simulink model "rcos_1"  (R2019b)
settings: Solver=VariableStepAuto  StartTime=0.0  StopTime=5e-3  RelTol=1e-3
values from neighbouring files (symbols this model uses):
  filter = rcosdesign(alpha,symNum,sym,'sqrt')    [loopFil.m]
libraries: dspsrcs4 x1
settings Model: Creator=Administrator  LastModifiedBy=Administrator

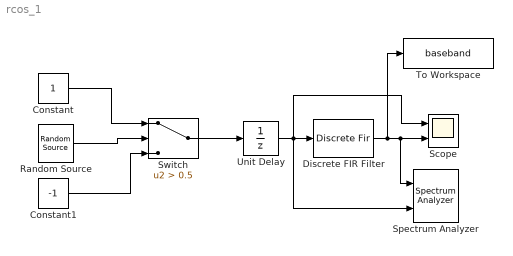
== system rcos_1 ==
  Constant : Constant  SampleTime=1/(6*19.2e3)
  Constant1 : Constant  Value=-1  SampleTime=1/(6*19.2e3)
  Discrete FIR Filter : DiscreteFir  Coefficients=filter(2,:)
  Random Source : dspsrcs4/Random Source  SrcType=Uniform  NormMethod=Ziggurat  CltLength=12  MinVal=0  MaxVal=1  MeanVal=0  VarVal=1  RepMode=Not repeatable  rawSeed=1  IsInherit=off  SampMode=Discrete  SampTime=1/(19.2e3)  SampFrame=1  DataType=Double  OutComplex=Real  OutputFrames=off
  Scope : Scope  NumInputPorts=2
  Spectrum Analyzer : SpectrumAnalyzer  NumInputPorts=2
  Switch : Switch  Criteria=u2 > Threshold  Threshold=0.5
  To Workspace : ToWorkspace  VariableName=baseband  SaveFormat=Timeseries  SampleTime=-1
  Unit Delay : UnitDelay  SampleTime=-1  HasFrameUpgradeWarning=on
  wires:
  Constant/1 -> Switch/1
  Constant1/1 -> Switch/3
  Random Source/1 -> Switch/2
  Switch/1 -> Unit Delay/1
  Unit Delay/1 -> Spectrum Analyzer/2, Scope/1, Discrete FIR Filter/1
  Discrete FIR Filter/1 -> Spectrum Analyzer/1, Scope/2, To Workspace/1
